simulink model "Simulink_U82KV100_jw"  (R2023a)
settings: Solver=FixedStepAuto  StartTime=0.0  StopTime=Inf  FixedStep=0.000625  RelTol=1e-3  EnableMultiTasking=on
undefined symbols (not defined in the file): square
libraries: c280xlib x5, c2000lib x1, simulink x1
settings Model: SimulationMode=external  ExtModeTrigDuration=8  Creator=RIMLAB  LastModifiedBy=RIMLAB
settings OptimizationCC: DefaultUnderspecifiedDataType=single  EnhancedBackFolding=on  PassReuseOutputArgsAs=Individual arguments  MaxStackSize=1024  OptimizeBlockOrder=speed  DifferentSizesBufferReuse=on  OptimizationCustomize=off  DenormalBehavior=FlushToZero  EfficientTunableParamExpr=on
settings DebuggingCC: MultiTaskDSMMsg=none  ParameterTunabilityLossMsg=error
settings HardwareCC: ProdBitPerChar=16  ProdBitPerInt=16  ProdBitPerPointer=32  ProdBitPerSizeT=32  ProdBitPerPtrDiffT=32  ProdLargestAtomicInteger=Integer  ProdLargestAtomicFloat=None  ProdWordSize=16  ProdLongLongMode=on  ProdHWDeviceType=Texas Instruments->C2000
settings ModelReferenceCC: ModelReferenceNumInstancesAllowed=Single
settings SFSimCC: MATLABDynamicMemAlloc=off
settings RTWCC: Description=Embedded Coder  SystemTargetFile=ert.tlc  HardwareBoard=TI Delfino F28379D LaunchPad  TemplateMakefile=ert_default_tmf  Toolchain=Texas Instruments Code Composer Studio (C2000)
settings CodeAppCC: ForceParamTrailComments=on  IgnoreCustomStorageClasses=off  OperatorAnnotations=on  SimulinkDataObjDesc=on  SFDataObjDesc=on  InsertBlockDesc=on
settings ERTTargetCC: CodeReplacementLibrary=TI C28x  SupportContinuousTime=on  ExtMode=on  ExtModeTransport=4  ExtModeStaticAlloc=on  ExtModeAutomaticAllocSize=off  ExtModeMexFile=ext_xcp  ExtModeMexArgs=1 23 5000000  ExtModeIntrfLevel=Level2 - Open

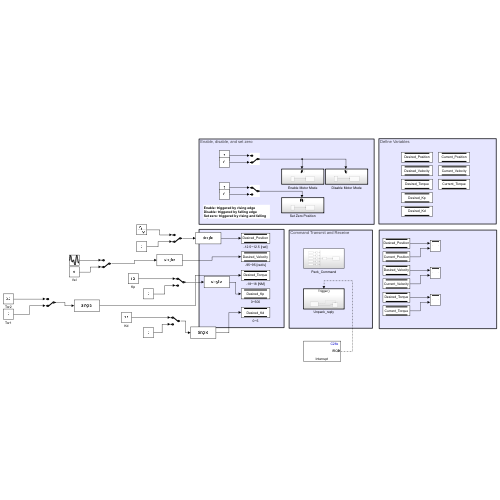
[thumbnail: Simulink's stored preview of the top-level diagram]
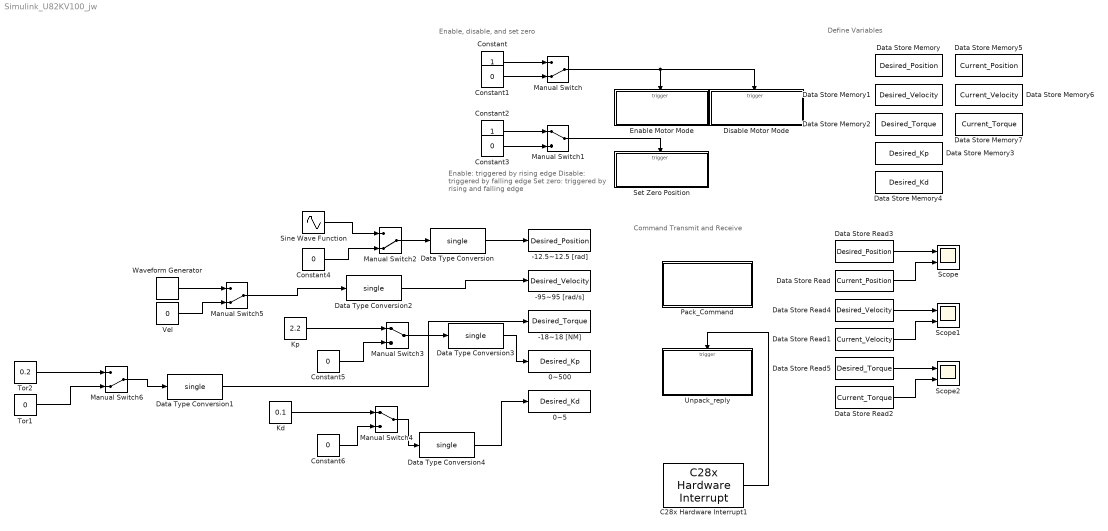
== system Simulink_U82KV100_jw ==
  note: Enable: triggered by rising edge
      | Disable: triggered by falling edge
      | Set zero: triggered by rising and falling edge
  note: Command Transmit and Receive
  note: Enable, disable, and set zero
  note: Define Variables
  -12.5~12.5 [rad] : DataStoreWrite  DataStoreName=Desired_Position  IndexOptions=Index vector (dialog)  Indices=1  OutputSizes=1
  -18~18 [NM] : DataStoreWrite  DataStoreName=Desired_Torque  IndexOptions=Index vector (dialog)  Indices=1  OutputSizes=1
  -95~95 [rad/s] : DataStoreWrite  DataStoreName=Desired_Velocity  IndexOptions=Index vector (dialog)  Indices=1  OutputSizes=1
  0~5 : DataStoreWrite  DataStoreName=Desired_Kd  IndexOptions=Index vector (dialog)  Indices=1  OutputSizes=1
  0~500 : DataStoreWrite  DataStoreName=Desired_Kp  IndexOptions=Index vector (dialog)  Indices=1  OutputSizes=1
  C28x Hardware Interrupt1 : c2000lib/Scheduling/C28x Hardware Interrupt  irqnumbers=[9]  pienumbers=[8]  irqpriorities=[30]  irqpreempts=[1]  showinput=off  dspchiptype=C280X
  Constant : Constant
  Constant1 : Constant  Value=0
  Constant2 : Constant
  Constant3 : Constant  Value=0
  Constant4 : Constant  Value=0
  Constant5 : Constant  Value=0  OutDataTypeStr=single
  Constant6 : Constant  Value=0  OutDataTypeStr=single
  Data Store Memory : DataStoreMemory  DataStoreName=Desired_Position  WriteAfterWriteMsg=warning  ShowAdditionalParam=off  OutDataTypeStr=single
  Data Store Memory1 : DataStoreMemory  DataStoreName=Desired_Velocity  WriteAfterWriteMsg=warning  ShowAdditionalParam=off  OutDataTypeStr=single
  Data Store Memory2 : DataStoreMemory  DataStoreName=Desired_Torque  WriteAfterWriteMsg=warning  ShowAdditionalParam=off  OutDataTypeStr=single
  Data Store Memory3 : DataStoreMemory  DataStoreName=Desired_Kp  WriteAfterWriteMsg=warning  ShowAdditionalParam=off  OutDataTypeStr=single
  Data Store Memory4 : DataStoreMemory  DataStoreName=Desired_Kd  WriteAfterWriteMsg=warning  ShowAdditionalParam=off  OutDataTypeStr=single
  Data Store Memory5 : DataStoreMemory  DataStoreName=Current_Position  WriteAfterWriteMsg=warning  ShowAdditionalParam=off  OutDataTypeStr=single
  Data Store Memory6 : DataStoreMemory  DataStoreName=Current_Velocity  WriteAfterWriteMsg=warning  ShowAdditionalParam=off  OutDataTypeStr=single
  Data Store Memory7 : DataStoreMemory  DataStoreName=Current_Torque  WriteAfterWriteMsg=warning  ShowAdditionalParam=off  OutDataTypeStr=single
  Data Store Read : DataStoreRead  DataStoreName=Current_Position  IndexOptions=Index vector (dialog)  Indices=1  OutputSizes=1
  Data Store Read1 : DataStoreRead  DataStoreName=Current_Velocity  IndexOptions=Index vector (dialog)  Indices=1  OutputSizes=1
  Data Store Read2 : DataStoreRead  DataStoreName=Current_Torque  IndexOptions=Index vector (dialog)  Indices=1  OutputSizes=1
  Data Store Read3 : DataStoreRead  DataStoreName=Desired_Position  IndexOptions=Index vector (dialog)  Indices=1  OutputSizes=1
  Data Store Read4 : DataStoreRead  DataStoreName=Desired_Velocity  IndexOptions=Index vector (dialog)  Indices=1  OutputSizes=1
  Data Store Read5 : DataStoreRead  DataStoreName=Desired_Torque  IndexOptions=Index vector (dialog)  Indices=1  OutputSizes=1
  Data Type Conversion{,1..4} (5 alike) : DataTypeConversion  OutDataTypeStr=single  SaturateOnIntegerOverflow=off  RndMeth=Floor
  Disable Motor Mode : Subsystem
  Enable Motor Mode : Subsystem
  Kd : Constant  Value=0.1  OutDataTypeStr=single  SampleTime=-1
  Kp : Constant  Value=2.2  OutDataTypeStr=single  SampleTime=-1
  Manual Switch{,2,5..6} (4 alike) : ManualSwitch  CurrentSetting=0
  Manual Switch1 : ManualSwitch
  Manual Switch3 : ManualSwitch
  Manual Switch4 : ManualSwitch
  Pack_Command : Subsystem
  Scope : Scope  NumInputPorts=2
  Scope1 : Scope  NumInputPorts=2
  Scope2 : Scope  NumInputPorts=2
  Set Zero Position : Subsystem
  Sine Wave Function : Sin  Amplitude=6.283185307  Frequency=3  SampleTime=0
  Tor1 : Constant  Value=0  OutDataTypeStr=single  SampleTime=-1
  Tor2 : Constant  Value=0.2  OutDataTypeStr=single  SampleTime=-1
  Unpack_reply : Subsystem
  Vel : Constant  Value=0  OutDataTypeStr=single  SampleTime=-1
  Waveform Generator : simulink/Sources/Waveform Generator  OutMin=[]  OutMax=[]  OutDataTypeStr=single  SelectedSignal=1  Signals=square('Amplitude',12,'Frequency',2,'Phase',0)  BlockNames=MultiportSwitch_ecbaca9dda044db  SampleTime=-1
  wires:
  Constant/1 -> Manual Switch/1
  Manual Switch/1 -> Enable Motor Mode/Trigger, Disable Motor Mode/Trigger
  Constant1/1 -> Manual Switch/2
  Constant2/1 -> Manual Switch1/1
  Constant3/1 -> Manual Switch1/2
  Manual Switch1/1 -> Set Zero Position/Trigger
  Data Type Conversion1/1 -> -18~18 [NM]/1
  Data Store Read3/1 -> Scope/1
  Data Store Read/1 -> Scope/2
  Data Store Read4/1 -> Scope1/1
  Data Store Read1/1 -> Scope1/2
  Data Store Read5/1 -> Scope2/1
  Data Store Read2/1 -> Scope2/2
  Data Type Conversion/1 -> -12.5~12.5 [rad]/1
  Manual Switch2/1 -> Data Type Conversion/1
  Constant4/1 -> Manual Switch2/2
  Constant5/1 -> Manual Switch3/2
  Constant6/1 -> Manual Switch4/2
  Vel/1 -> Manual Switch5/2
  Tor2/1 -> Manual Switch6/1
  Tor1/1 -> Manual Switch6/2
  Manual Switch6/1 -> Data Type Conversion1/1
  Manual Switch5/1 -> Data Type Conversion2/1
  Data Type Conversion2/1 -> -95~95 [rad/s]/1
  Manual Switch3/1 -> Data Type Conversion3/1
  Data Type Conversion3/1 -> 0~500/1
  Kp/1 -> Manual Switch3/1
  Kd/1 -> Manual Switch4/1
  Manual Switch4/1 -> Data Type Conversion4/1
  Data Type Conversion4/1 -> 0~5/1
  Waveform Generator/1 -> Manual Switch5/1
  Sine Wave Function/1 -> Manual Switch2/1
  C28x Hardware Interrupt1/1 -> Unpack_reply/Trigger

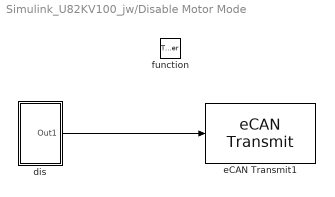
== system Simulink_U82KV100_jw/Disable Motor Mode ==
  function : TriggerPort  TriggerType=falling  VariantControl=(inherit)
  dis : Subsystem
  eCAN Transmit1 : c280xlib/eCAN Transmit  chipFamily=C280x  useModule=eCAN_B  mailboxNo=1  messageID=1  messageType=Standard (11-bit identifier)  enableBlockingMode=off  postInterrupt=off  interruptLine=0
      settings: LibrarySourceBlock=c2837xDlib/eCAN Transmit
  wires:
  dis/1(Out1) -> eCAN Transmit1/1

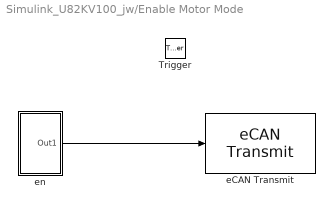
== system Simulink_U82KV100_jw/Enable Motor Mode ==
  Trigger : TriggerPort  VariantControl=(inherit)  PortDimensions=1
  eCAN Transmit : c280xlib/eCAN Transmit  chipFamily=C280x  useModule=eCAN_B  mailboxNo=1  messageID=1  messageType=Standard (11-bit identifier)  enableBlockingMode=off  postInterrupt=off  interruptLine=0
      settings: LibrarySourceBlock=c2837xDlib/eCAN Transmit
  en : Subsystem
  wires:
  en/1(Out1) -> eCAN Transmit/1

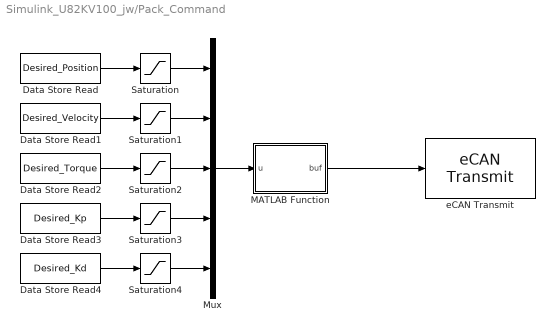
== system Simulink_U82KV100_jw/Pack_Command ==
  Data Store Read : DataStoreRead  DataStoreName=Desired_Position  IndexOptions=Index vector (dialog)  Indices=1  OutputSizes=1
  Data Store Read1 : DataStoreRead  DataStoreName=Desired_Velocity  IndexOptions=Index vector (dialog)  Indices=1  OutputSizes=1
  Data Store Read2 : DataStoreRead  DataStoreName=Desired_Torque  IndexOptions=Index vector (dialog)  Indices=1  OutputSizes=1
  Data Store Read3 : DataStoreRead  DataStoreName=Desired_Kp  IndexOptions=Index vector (dialog)  Indices=1  OutputSizes=1
  Data Store Read4 : DataStoreRead  DataStoreName=Desired_Kd  IndexOptions=Index vector (dialog)  Indices=1  OutputSizes=1
  MATLAB Function : MATLAB Function  TreatAsAtomicUnit=on
  Mux : Mux  Inputs=5
  Saturation : Saturate  UpperLimit=12.5  LowerLimit=-12.5
  Saturation1 : Saturate  UpperLimit=95  LowerLimit=-95
  Saturation2 : Saturate  UpperLimit=18  LowerLimit=-18
  Saturation3 : Saturate  UpperLimit=500  LowerLimit=0
  Saturation4 : Saturate  UpperLimit=5  LowerLimit=0
  eCAN Transmit : c280xlib/eCAN Transmit  chipFamily=C280x  useModule=eCAN_B  mailboxNo=1  messageID=1  messageType=Standard (11-bit identifier)  enableBlockingMode=off  postInterrupt=off  interruptLine=0
      settings: LibrarySourceBlock=c2837xDlib/eCAN Transmit
  wires:
  Data Store Read/1 -> Saturation/1
  Data Store Read1/1 -> Saturation1/1
  Data Store Read2/1 -> Saturation2/1
  Data Store Read3/1 -> Saturation3/1
  Data Store Read4/1 -> Saturation4/1
  Saturation/1 -> Mux/1
  Saturation1/1 -> Mux/2
  Saturation2/1 -> Mux/3
  Saturation3/1 -> Mux/4
  Saturation4/1 -> Mux/5
  Mux/1 -> MATLAB Function/1(u)
  MATLAB Function/1(buf) -> eCAN Transmit/1

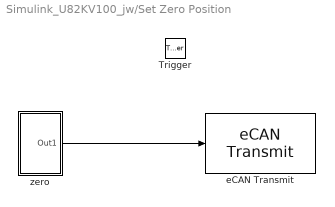
== system Simulink_U82KV100_jw/Set Zero Position ==
  Trigger : TriggerPort  TriggerType=either  VariantControl=(inherit)  PortDimensions=1
  eCAN Transmit : c280xlib/eCAN Transmit  chipFamily=C280x  useModule=eCAN_B  mailboxNo=1  messageID=1  messageType=Standard (11-bit identifier)  enableBlockingMode=off  postInterrupt=off  interruptLine=0
      settings: LibrarySourceBlock=c2837xDlib/eCAN Transmit
  zero : Subsystem
  wires:
  zero/1(Out1) -> eCAN Transmit/1

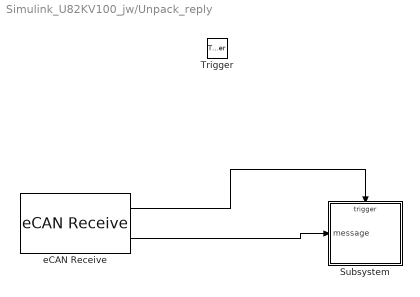
== system Simulink_U82KV100_jw/Unpack_reply ==
  Trigger : TriggerPort  TriggerType=function-call  VariantControl=(inherit)  PortDimensions=1
  Subsystem : Subsystem
  eCAN Receive : c280xlib/eCAN Receive  chipFamily=C280x  useModule=eCAN_B  mailboxNo=0  messageID=0  messageType=Standard (11-bit identifier)  enableAcceptanceFiltering=on  messageIDMask=bin2dec('00000000001')  sampleTime=-1  dataType=uint8  outputAction=Output last received values  initValue=0  outputMessageID=off  outputMessageLength=off  outputMessageTimeStamp=off  postInterrupt=on  interruptLine=1
      settings: LibrarySourceBlock=c2837xDlib/eCAN Receive
  wires:
  eCAN Receive/2 -> Subsystem/1(message)
  eCAN Receive/1 -> Subsystem/Trigger

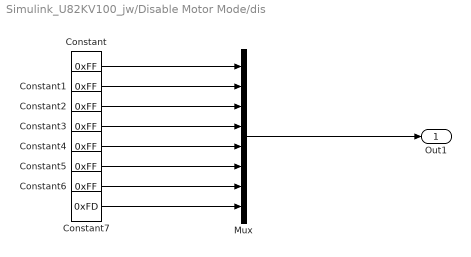
== system Simulink_U82KV100_jw/Disable Motor Mode/dis ==
  Constant{,1..6} (7 alike) : Constant  Value=0xFF  SampleTime=-1
  Constant7 : Constant  Value=0xFD  SampleTime=-1
  Mux : Mux  Inputs=8
  Out1 : Outport
  wires:
  Mux/1 -> Out1/1
  Constant4/1 -> Mux/5
  Constant1/1 -> Mux/2
  Constant3/1 -> Mux/4
  Constant5/1 -> Mux/6
  Constant/1 -> Mux/1
  Constant6/1 -> Mux/7
  Constant2/1 -> Mux/3
  Constant7/1 -> Mux/8

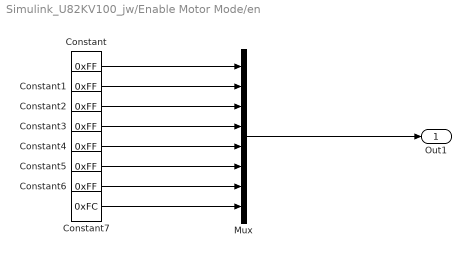
== system Simulink_U82KV100_jw/Enable Motor Mode/en ==
  Constant{,1..6} (7 alike) : Constant  Value=0xFF  SampleTime=-1
  Constant7 : Constant  Value=0xFC  SampleTime=-1
  Mux : Mux  Inputs=8
  Out1 : Outport
  wires:
  Constant7/1 -> Mux/8
  Constant2/1 -> Mux/3
  Constant6/1 -> Mux/7
  Constant/1 -> Mux/1
  Constant5/1 -> Mux/6
  Constant3/1 -> Mux/4
  Constant1/1 -> Mux/2
  Constant4/1 -> Mux/5
  Mux/1 -> Out1/1

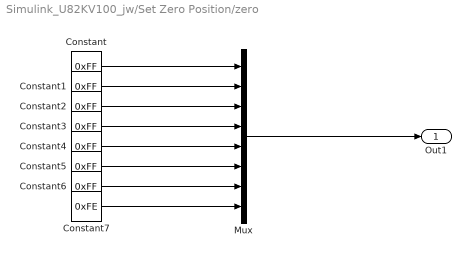
== system Simulink_U82KV100_jw/Set Zero Position/zero ==
  Constant{,1..6} (7 alike) : Constant  Value=0xFF  SampleTime=-1
  Constant7 : Constant  Value=0xFE  SampleTime=-1
  Mux : Mux  Inputs=8
  Out1 : Outport
  wires:
  Mux/1 -> Out1/1
  Constant4/1 -> Mux/5
  Constant1/1 -> Mux/2
  Constant3/1 -> Mux/4
  Constant5/1 -> Mux/6
  Constant/1 -> Mux/1
  Constant6/1 -> Mux/7
  Constant2/1 -> Mux/3
  Constant7/1 -> Mux/8

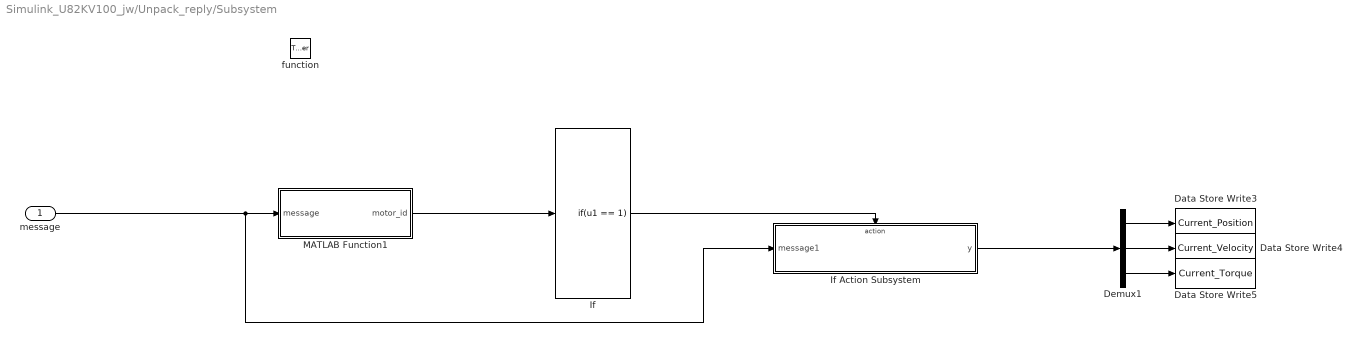
== system Simulink_U82KV100_jw/Unpack_reply/Subsystem ==
  message : Inport
  function : TriggerPort  TriggerType=function-call  VariantControl=(inherit)
  Data Store Write3 : DataStoreWrite  DataStoreName=Current_Position  IndexOptions=Index vector (dialog)  Indices=1  OutputSizes=1
  Data Store Write4 : DataStoreWrite  DataStoreName=Current_Velocity  IndexOptions=Index vector (dialog)  Indices=1  OutputSizes=1
  Data Store Write5 : DataStoreWrite  DataStoreName=Current_Torque  IndexOptions=Index vector (dialog)  Indices=1  OutputSizes=1
  Demux1 : Demux  Outputs=3
  If : If  IfExpression=u1 == 1  ShowElse=off
  If Action Subsystem : Subsystem  TreatAsAtomicUnit=on
  MATLAB Function1 : MATLAB Function  TreatAsAtomicUnit=on
  wires:
  message/1 -> MATLAB Function1/1(message), If Action Subsystem/1(message1)
  MATLAB Function1/1(motor_id) -> If/1
  If/1 -> If Action Subsystem/Action
  Demux1/2 -> Data Store Write4/1
  If Action Subsystem/1(y) -> Demux1/1
  Demux1/1 -> Data Store Write3/1
  Demux1/3 -> Data Store Write5/1

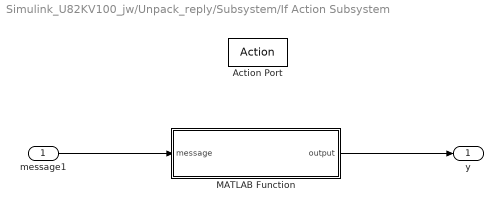
== system Simulink_U82KV100_jw/Unpack_reply/Subsystem/If Action Subsystem ==
  message1 : Inport
  Action Port : ActionPort  ActionPortLabel=if(u1 == 1)
  MATLAB Function : MATLAB Function  TreatAsAtomicUnit=on
  y : Outport
  wires:
  message1/1 -> MATLAB Function/1(message)
  MATLAB Function/1(output) -> y/1

== matlab function Simulink_U82KV100_jw/Unpack_reply/Subsystem/MATLAB Function1 ==
  data: message input; motor_id output
function motor_id = fcn(message)
message = uint16(message);
motor_id = message(1);

== matlab function Simulink_U82KV100_jw/Unpack_reply/Subsystem/If Action Subsystem/MATLAB Function ==
  data: message input; output output
function output  = fcn(message)
output = single(zeros(1,3));
message = uint16(message);
uintpos = bitor(bitshift(message(2),8,'uint16'),message(3),'uint16');
uintvel = bitor(bitshift(message(4),4,'uint16'), bitshift(message(5),-4,'uint16'),'uint16');
tintvel = bitor(bitshift(bitand(message(5),uint16(15),'uint16'),8,'uint16') , message(6),'uint16');

output(1) = single(uintpos)*25/65535.0 -12.5;
output(2) = single(uintvel)*190/4095.0 -95;
output(3) = single(tintvel)*36/4095.0 -18;

== matlab function Simulink_U82KV100_jw/Pack_Command/MATLAB Function ==
  data: u input; buf output
function buf  = fcn(u)
buf = uint8(zeros(1,8));
upos = uint16(((u(1)+12.5)*65535.0/25));
uvel = uint16(((u(2)+95)*4095.0/190));
utor = uint16(((u(3)+18)*4095.0/36));
ukp = uint16(((u(4))*4095.0/500));
ukd = uint16(((u(5))*4095.0/5));

buf(1) = bitshift(upos,-8,'uint16');                                       
buf(2) = bitand(upos, uint16(255),'uint16');   
buf(3) = bitshift(uvel,-4,'uint16');
buf(4) = bitor(bitshift(bitand(uvel, uint16(15),'uint16'),4,'uint16'), bitshift(ukp,-8,'uint16'),'uint16');
buf(5) = bitand(ukp, uint16(255),'uint16');
buf(6) = bitshift(ukd,-4,'uint16');
buf(7) = bitor(bitshift(bitand(ukd , uint16(15),'uint16'),4,'uint16'), bitshift(utor,-8,'uint16'),'uint16');
buf(8) = bitand(utor, uint16(255),'uint16');
